simulink model "MPPT_with_INC"  (R2022a)
settings: Solver=ode23tb  StartTime=0.0  StopTime=5  RelTol=1e-3
libraries: spsSeriesRLCBranchLib x4, spsDCVoltageSourceLib x1, spsDiodeLib x1, spsCurrentMeasurementLib x1, spsMosfetLib x1, spsPVArrayLib x1, spsPWMGeneratorDCDCLib x1, eeStairGenerator x1, spsVoltageMeasurementLib x1, spspowerguiLib x1
settings Model: Creator=Sajid Ali  LastModifiedBy=Sajid Ali
settings OptimizationCC: OptimizeBlockIOStorage=off  OptimizeDataStoreBuffers=off  BusAssignmentInplaceUpdate=off
settings DebuggingCC: SFUnexpectedBacktrackingDiag=warning  SFNoUnconditionalDefaultTransitionDiag=warning
settings RTWCC: GenerateReport=on  BuildConfiguration=Debug  LaunchReport=on
settings CodeAppCC: ForceParamTrailComments=on  MATLABSourceComments=on  EnableCustomComments=on
settings GRTTargetCC: CombineSignalStateStructs=on  SupportVariableSizeSignals=on  MultiInstanceErrorCode=Warning

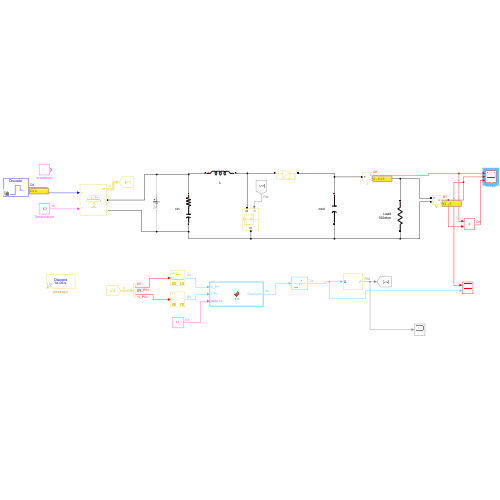
[thumbnail: Simulink's stored preview of the top-level diagram]
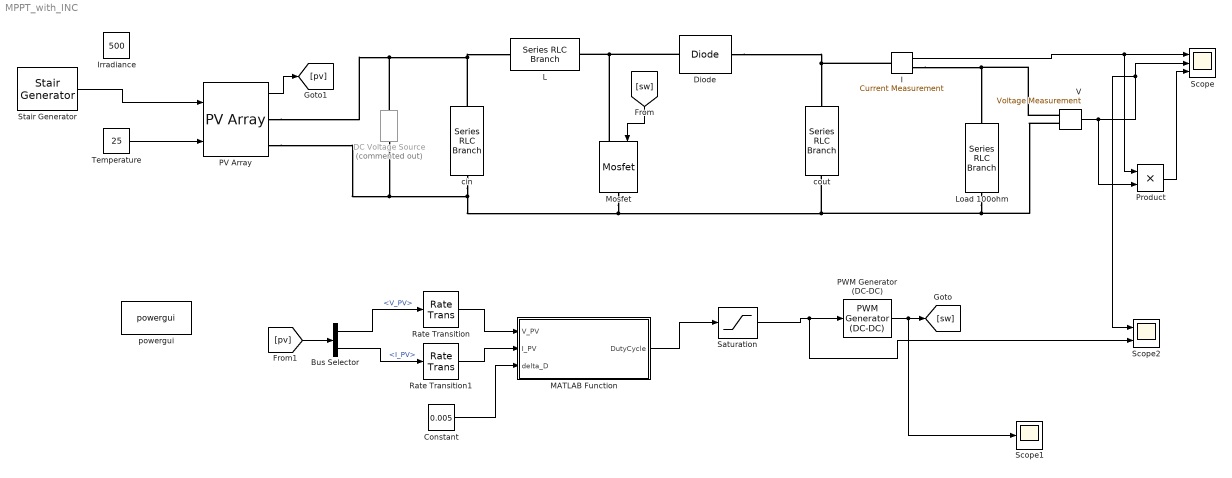
== system MPPT_with_INC ==
  Bus Selector : BusSelector  OutputSignals=V_PV,I_PV
  Constant : Constant  Value=0.005
  DC Voltage Source : spsDCVoltageSourceLib/DC Voltage Source  Commented=on  Amplitude=12  Measurements=None
  Diode : spsDiodeLib/Diode  Ron=0.001  Lon=0  Vf=0.8  IC=0  UseSnubber=0  Rs=500  Cs=250e-9  Measurements=off
  I : spsCurrentMeasurementLib/Current Measurement  PhasorSimulation=off  OutputType=Complex  PSBequivalent=0
  Irradiance : Constant  Value=500
  L : spsSeriesRLCBranchLib/Series RLC Branch  LConnTagsString=__new0  RConnTagsString=__new0  BranchType=L  Resistance=1  Inductance=700e-6  SetiL0=off  InitialCurrent=0  Capacitance=100e-6  Setx0=off  InitialVoltage=0  Measurements=None
  Load 100ohm : spsSeriesRLCBranchLib/Series RLC Branch  LConnTagsString=__new0  RConnTagsString=__new0  BranchType=R  Resistance=100  Inductance=1e-3  SetiL0=off  InitialCurrent=0  Capacitance=100e-6  Setx0=off  InitialVoltage=0  Measurements=None
  MATLAB Function : MATLAB Function  TreatAsAtomicUnit=on
  Mosfet : spsMosfetLib/Mosfet  Ron=0.1  Lon=0  Rd=0.01  Vfd=0  IC=0  Rs=1e5  Cs=inf  Measurements=off
  PV Array : spsPVArrayLib/PV Array  Npar=1  Nser=1  PlotType=array @ 1000 W/m2 & specified temperatures  S_vec="[ 1000  500  100 ]"  Temp_C_vec="[ 45 25  ]"  ModuleName=User-defined  PlotWhenSelected=off  Pm=102.09  Ncell=60  Voc=29  Isc=4.5  Vm=24.9  Im=4.1  beta_Voc_pc=-0.36099  alpha_Isc_pc=0.102  beta_Voc=-0.10469  alpha_Isc=0.00459  IL=4.5032  I0=1.6559e-10  nI=0.7848  Rsh=119.4993  Rs=0.085247  RobustModel=off  RobustCellTemperature=313.3991  BAL=on  Tc=1e-6  Tfilter=5e-5
  PWM Generator (DC-DC) : spsPWMGeneratorDCDCLib/PWM Generator (DC-DC)  Fsw=62.5e3  Ts=0
  Product : Product
  Rate Transition : RateTransition  OutPortSampleTime=1
  Rate Transition1 : RateTransition  OutPortSampleTime=1
  Saturation : Saturate  UpperLimit=0.9  LowerLimit=0.1
  Scope : Scope  NumInputPorts=3
  Scope1 : Scope
  Scope2 : Scope  NumInputPorts=2
  Stair Generator : eeStairGenerator/Stair Generator  LabelModeActiveChoice=Discrete  TimeInput=[0 1 2 3 4 5 ]  AmplitudeInput=[500 500 700 700 600 600]  SampleTime=1/100  RepeatPattern=off  OutDataTypeStr=double
      settings: SourceProductBaseCode=PS
  Temperature : Constant  Value=25
  V : spsVoltageMeasurementLib/Voltage Measurement  PhasorSimulation=off  OutputType=Complex  PSBequivalent=0
  cin : spsSeriesRLCBranchLib/Series RLC Branch  LConnTagsString=__new0  RConnTagsString=__new0  BranchType=RC  Resistance=1e-3  Inductance=1e-3  SetiL0=off  InitialCurrent=0  Capacitance=100e-6  Setx0=off  InitialVoltage=0  Measurements=None
  cout : spsSeriesRLCBranchLib/Series RLC Branch  LConnTagsString=__new0  RConnTagsString=__new0  BranchType=C  Resistance=1  Inductance=1e-3  SetiL0=off  InitialCurrent=0  Capacitance=100e-6  Setx0=off  InitialVoltage=0  Measurements=None
  powergui : spspowerguiLib/powergui  Priority=1  SimulationMode=Discrete  SampleTime=1e-6  frequency=60  Iterations=50  frequencyindice=0  Pbase=100e6  ErrMax=1e-4  UnitsV=kV  UnitsW=MW  buscounter=0  FunctionMessages=off  echomessages=off  EnableUseOfTLC=off  CurrentSourceSwitches=off  DisableSnubberDevices=off  DisableRonSwitches=off  DisableVfSwitches=off  DisplayEquations=off  AutomaticDiscreteSolvers=off  SolverType=Tustin/Backward Euler (TBE)  Interpol=off  ExternalGateDelay=off  methode=off  Ts=100  x0status=blocks  SPID=on  SwTol=0  HookPort=off  NonlinearTolerance=1e-4  nMaxIteration=100  ContinueOnMaxIteration=off  RestoreLinks=warning  ResistiveCurrentMeasurement=off  Frange=[0:2:500]  Ylog=off  Xlog=on  ShowGrid=off  save=off  variable=ZData  structure=0  ZoomFFT=off  StartTime=0.0  cycles=1  DisplayStyle=1  fundamental=60  FreqAxis=off  MaxFrequency=1000  frequencyindicesteady=1  RmsSteady=1  display=off
  wires:
  [sw] -> Mosfet/1
  PV Array/1 -> [pv]
  Stair Generator/1 -> PV Array/1
  Temperature/1 -> PV Array/2
  [pv] -> Bus Selector/1
  I/1 -> Product/1, Scope/1
  V/1 -> Product/2, Scope2/1, Scope/2
  MATLAB Function/1(DutyCycle) -> Saturation/1
  PWM Generator (DC-DC)/1 -> [sw], Scope1/1
  Bus Selector/1 -> Rate Transition/1  "<V_PV>"
  Bus Selector/2 -> Rate Transition1/1  "<I_PV>"
  Rate Transition/1 -> MATLAB Function/1(V_PV)
  Rate Transition1/1 -> MATLAB Function/2(I_PV)
  Constant/1 -> MATLAB Function/3(delta_D)
  Product/1 -> Scope/3
  Saturation/1 -> Scope2/2, PWM Generator (DC-DC)/1
  connections:
  Diode/LConn1 -- Mosfet/LConn1 -- L/RConn1
  Diode/RConn1 -- I/LConn1 -- cout/LConn1
  I/RConn1 -- Load 100ohm/LConn1 -- V/LConn1
  V/LConn2 -- Load 100ohm/RConn1 -- DC Voltage Source/LConn1 -- PV Array/RConn2 -- cin/RConn1 -- Mosfet/RConn1 -- cout/RConn1
  cin/LConn1 -- DC Voltage Source/RConn1 -- PV Array/RConn1 -- L/LConn1

== matlab function MPPT_with_INC/MATLAB Function ==
  data: V_PV input; DutyCycle output; I_PV input; delta_D input
function DutyCycle = fcn(V_PV, I_PV,delta_D)





% %%____________________P&O___________________
% persistent V_PV_1 P_PV_1 D;   % global variable declaration 
% 
% % Variable initialization
% if(isempty(V_PV_1))
%     V_PV_1=0;
%     P_PV_1=0;
%     D=0.5;
%     %%disp("initialized")
% end


%MPPT algorithm P&O
% P_PV=V_PV*I_PV;
% 
% if(P_PV-P_PV_1~=0)
% 
%     if(P_PV-P_PV_1>0)
%         if(V_PV-V_PV_1>0)
%             D=D+delta_D;
%         else
%             D=D-delta_D;
%         end
%     else
%         if(V_PV-V_PV_1>0)
%             D=D-delta_D;
%         else
%             D=D+delta_D;
%         end
%     
%     end
% 
% end



% 
% %set previous values
% V_PV_1=V_PV;
% P_PV_1=P_PV;
% 
% DutyCycle=D;
%_______________________________End P&O ___________________________


%%MPPT algorithm INC


persistent V_PV_1 I_PV_1 D;   % global variable declaration 

% Variable initialization
if(isempty(V_PV_1))
    V_PV_1=0;
    I_PV_1=0;
    D=0.5;
    %%disp("initialized")
end


dV=V_PV-V_PV_1;
if (dV==0)
    dV=1e-5;
end
dI=I_PV-I_PV_1;

if(dV==0)
	if(dI==0)
	%return
	else
		if(dI>0)
			D=D+delta_D;%increase voltage
		else
			D=D-delta_D;%decrease voltage
		end
	end	
else
if(I_PV+(dI/dV)*V_PV==0)
	%return	
else
	if(I_PV+(dI/dV)*V_PV>0)
		D=D-delta_D;%decrease voltage
	else
		D=D+delta_D;%increase voltage
	end

end
end
V_PV_1=V_PV;
I_PV_1=I_PV;

DutyCycle=D;
